simulink model "steer_model_pt1_pt2DeadTime_comparison"  (R2017a)
settings: Solver=FixedStepAuto  StartTime=0.0  StopTime=10.0  FixedStep=1e-2  RelTol=1e-3
settings Model: Creator=ilja  LastModifiedBy=ilja

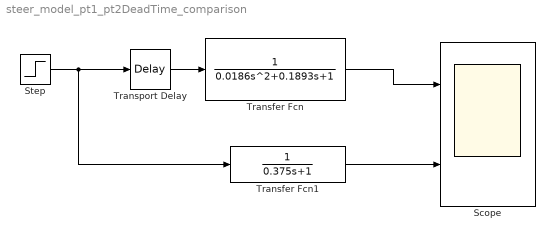
== system steer_model_pt1_pt2DeadTime_comparison ==
  Scope : Scope  NumInputPorts=2
  Step : Step  SampleTime=0
  Transfer Fcn : TransferFcn  Denominator=[0.0186 0.1893 1]
  Transfer Fcn1 : TransferFcn  Denominator=[0.375 1]
  Transport Delay : TransportDelay  DelayTime=0.2
  wires:
  Transfer Fcn1/1 -> Scope/2
  Transfer Fcn/1 -> Scope/1
  Step/1 -> Transport Delay/1, Transfer Fcn1/1
  Transport Delay/1 -> Transfer Fcn/1
